simulink model "GPS1_Kvaser_R2018a_v3_0719"  (R2018a)
settings: Solver=FixedStepAuto  StartTime=0.0  StopTime=inf  FixedStep=0.02  RelTol=1e-3
undefined symbols (not defined in the file): canChannel
libraries: dspinverses x11, canmsglib x6, canlib x4
(part 1 of 2)
settings Model: Creator=ZNYZY  LastModifiedBy=RickyFang
settings SFSimCC: SimUseLocalCustomCode=on
settings RTWCC: RTWUseLocalCustomCode=on

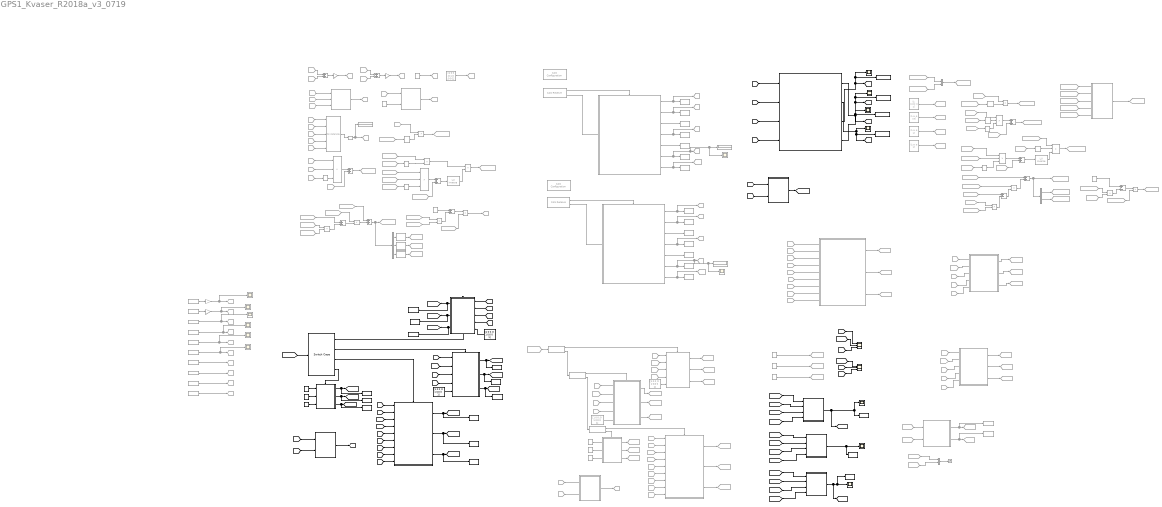
== system GPS1_Kvaser_R2018a_v3_0719 ==
  note: head要乘pi/180
  note: 离线仿真
  note: 试验设计
      | 1.双GPS走同一直线，改L值，反复3次
      | 2.双GPS贴在一起，改L值，反复3次
      | 3.双GPS走同一段曲线，改L值，反复3次
  note: 最终用于EKF卡尔曼滤波的观测速度
  note: dSPACE
  note: 通道1：GPS1的信号——取sate1、head1、lat1、long1、speed1
      | 通道2：GPS2的信号——取sate2、head2、lat2、long2、speed2
      | 通道3：车辆信号——取Vehicle_Speed、Acc_Ego
  note: EKF_mode = 3
  note: GPS测得车速与车身DBC的车速进行比较选择
  note: X_predict = A*X_optimal(:,i-1);
  note: EKF_mode=3，单GPS2工作；
      | EKF_mode=2，单GPS1工作；
      | EKF_mode=1，双GPS融合工作；
      | EKF_mode=0，不可测；
  note: 得到EKF的模式
  note: GPS经纬度坐标系转大地坐标系
  note: Kvaser读取GPS
  note: EKF_mode = 1
  note: EKF_mode = 2
  note: EKF_mode = 0
  note: EKF_mode = 3
  note: EKF_mode = 1
  note: EKF_mode = 0.1.2
  note: EKF_mode = 2
  note: EKF_mode = 1
  note: EKF_mode = 0
  note: EKF_mode判断逻辑
  note: EKF_mode判断逻辑
  " LU Inverse" : dspinverses/ LU Inverse  Commented=on
  " LU Inverse1" : dspinverses/ LU Inverse  Commented=on
  Add : Sum  Commented=on  Inputs=+-
  CAN Configuration : canlib/CAN Configuration  Commented=on  BlockHandle=4516.0012  Device=MathWorks Virtual 1 (Channel 1)  DeviceMenu=MathWorks Virtual 1 (Channel 1)  ObjConstructor=canChannel('MathWorks', 'Virtual 1', 1)  BusSpeed=500000  EnableBitParameters=off  AckMode=Normal
      settings: SourceProductBaseCode=VN
  CAN Configuration1 : canlib/CAN Configuration  Commented=on  BlockHandle=4517.0012  Device=MathWorks Virtual 1 (Channel 1)  DeviceMenu=MathWorks Virtual 1 (Channel 1)  ObjConstructor=canChannel('MathWorks', 'Virtual 1', 1)  BusSpeed=500000  EnableBitParameters=off  AckMode=Normal
      settings: SourceProductBaseCode=VN
  CAN Receive1 : canlib/CAN Receive  Commented=on  BlockHandle=4518.0012  Device=MathWorks Virtual 1 (Channel 1)  DeviceMenu=MathWorks Virtual 1 (Channel 1)  ObjConstructor=canChannel('MathWorks', 'Virtual 1', 1)  EnableStandardIDsFilter=off  StdIDsCombo=Allow all  StandardIDs=0  EnableExtendedIDsFilter=off  ExtIDsCombo=Allow all  ExtendedIDs=0  SampleTime=0.01  MsgsPerTimestep=all  InternalFilterUpdateStatus=on  BusOutput=off
      settings: SourceProductBaseCode=VN
  CAN Receive2 : canlib/CAN Receive  Commented=on  BlockHandle=4519.0012  Device=MathWorks Virtual 1 (Channel 1)  DeviceMenu=MathWorks Virtual 1 (Channel 1)  ObjConstructor=canChannel('MathWorks', 'Virtual 1', 1)  EnableStandardIDsFilter=off  StdIDsCombo=Allow all  StandardIDs=0  EnableExtendedIDsFilter=off  ExtIDsCombo=Allow all  ExtendedIDs=0  SampleTime=0.01  MsgsPerTimestep=all  InternalFilterUpdateStatus=on  BusOutput=off
      settings: SourceProductBaseCode=VN
  Constant : Constant  Commented=on  Value=[1 0 0 ;0 1 0 ;0 0 1]
  Constant1 : Constant  Commented=on  Value=0.01
  Constant{4..7,10..11} (6 alike) : Constant  Commented=on  Value=0
  Constant12 : Constant  Commented=on  Value=[1 0 0 ;0 1 0;0 0 1]
  Constant13 : Constant  Value=0
  Constant14 : Constant  Value=[1 0 0 ;0 1 0;0 0 1]
  Constant15 : Constant  Value=0
  Constant16 : Constant  Value=[1 0 0 ;0 1 0;0 0 1]
  Constant17 : Constant  Commented=on  Value=[1 0.02; 0 1]
  Constant18 : Constant  Commented=on  Value=[1 0; 0 10]
  Constant19 : Constant  Commented=on  Value=[1 0; 0 1]
  Constant2 : Constant  Commented=on  Value=0.3
  Constant20 : Constant  Commented=on  Value=[1 0; 0 1]
  Constant21 : Constant  Commented=on  Value=eye(2)
  Constant3 : Constant  Commented=on  Value=eye(3)
  Constant8 : Constant  Value=0
  Constant9 : Constant  Commented=on  Value=[1 0 0 ;0 1 0;0 0 1]
  Delay : Delay  Commented=on  DelayLength=1
  Delay1 : Delay  Commented=on  DelayLength=1
  Delay2 : Delay  Commented=on  DelayLength=1
  Demux : Demux  Commented=on  Outputs=3
  Demux1 : Demux  Commented=on  Outputs=2
  Display : Display  Commented=on
  Display1 : Display  Commented=on
  Display2 : Display  Commented=on
  EKF_HEAD : Scope
  EKF_HEAD_SUB : Subsystem
  EKF_LAT : Scope
  EKF_LAT_SUB : Subsystem
  EKF_LONG : Scope
  EKF_LONG_SUB : Subsystem
  From Workspace : FromWorkspace  Commented=on  VariableName=head1
  From Workspace1 : FromWorkspace  Commented=on  VariableName=head2
  From Workspace2 : FromWorkspace  Commented=on  VariableName=lat1
  From Workspace3 : FromWorkspace  Commented=on  VariableName=lat2
  From Workspace4 : FromWorkspace  Commented=on  VariableName=long1
  From Workspace5 : FromWorkspace  Commented=on  VariableName=long2
  From Workspace6 : FromWorkspace  Commented=on  VariableName=sate1
  From Workspace7 : FromWorkspace  Commented=on  VariableName=sate2
  From Workspace8 : FromWorkspace  Commented=on  VariableName=speed1
  From Workspace9 : FromWorkspace  Commented=on  VariableName=speed2
  From{10,15,18,65,77,133} (6 alike) : From  Commented=on  GotoTag=speed1
  From11 : From  Commented=on  GotoTag=long1
  From110 : From  Commented=on  GotoTag=Vehicle_Speed
  From111 : From  Commented=on  GotoTag=Acc_Ego
  From112 : From  Commented=on  GotoTag=X_optimal_vehicle
  From113 : From  Commented=on  GotoTag=A_Vehicle
  From114 : From  Commented=on  GotoTag=A_Vehicle
  From115 : From  Commented=on  GotoTag=A_Vehicle
  From116 : From  Commented=on  GotoTag=P_Vehicle
  From117 : From  Commented=on  GotoTag=Q_Vehicle
  From{118,120,122,127,130} (5 alike) : From  Commented=on  GotoTag=C_Vehicle
  From119 : From  Commented=on  GotoTag=P_predict_Vehicle
  From{9,12,16,73..74} (5 alike) : From  Commented=on  GotoTag=head1
  From121 : From  Commented=on  GotoTag=P_predict_Vehicle
  From123 : From  Commented=on  GotoTag=R_Vehicle
  From124 : From  Commented=on  GotoTag=X_predict_vehicle
  From125 : From  Commented=on  GotoTag=K_Vehicle
  From126 : From  Commented=on  GotoTag=Y_Vehicle
  From128 : From  Commented=on  GotoTag=X_predict_vehicle
  From129 : From  Commented=on  GotoTag=K_Vehicle
  From13 : From  Commented=on  GotoTag=long1
  From131 : From  Commented=on  GotoTag=P_predict_Vehicle
  From132 : From  Commented=on  GotoTag=KF_Vehicle_Speed
  From{19,50,54,61,69,134} (6 alike) : From  Commented=on  GotoTag=speed2
  From135 : From  Commented=on  GotoTag=sate1
  From136 : From  Commented=on  GotoTag=sate2
  From137 : From  Commented=on  GotoTag=EKF_lat
  From138 : From  Commented=on  GotoTag=EKF_long
  From139 : From  Commented=on  GotoTag=EKF_long_abs
  From14 : From  Commented=on  GotoTag=lat1
  From140 : From  Commented=on  GotoTag=EKF_lat_abs
  From{7,17,53,63,68} (5 alike) : From  Commented=on  GotoTag=head2
  From20 : From  Commented=on  GotoTag=y2
  From21 : From  Commented=on  GotoTag=y1
  From22 : From  Commented=on  GotoTag=x2
  From23 : From  Commented=on  GotoTag=x1
  From24 : From  Commented=on
  From25 : From  Commented=on  GotoTag=X_optimal
  From26 : From  Commented=on
  From27 : From  Commented=on  GotoTag=P
  From28 : From  Commented=on
  From29 : From  Commented=on  GotoTag=Q
  From30 : From  Commented=on  GotoTag=P_predict
  From{31..32,34,39,42} (5 alike) : From  Commented=on  GotoTag=C
  From33 : From  Commented=on  GotoTag=P_predict
  From{6,35,51,57,72} (5 alike) : From  Commented=on  GotoTag=R
  From36 : From  Commented=on  GotoTag=X_predict
  From37 : From  Commented=on  GotoTag=K
  From38 : From  Commented=on  GotoTag=Y
  From40 : From  Commented=on  GotoTag=X_predict
  From41 : From  Commented=on  GotoTag=K
  From43 : From  Commented=on  GotoTag=P_predict
  From44 : From  Commented=on  GotoTag=head
  From45 : From  Commented=on  GotoTag=speed
  From46 : From  Commented=on  GotoTag=T
  From47 : From  Commented=on  GotoTag=head
  From48 : From  Commented=on  GotoTag=head
  From49 : From  Commented=on  GotoTag=lat2
  From52 : From  Commented=on  GotoTag=lat1
  From55 : From  Commented=on  GotoTag=long2
  From56 : From  Commented=on  GotoTag=lat2
  From58 : From  Commented=on  GotoTag=x1
  From59 : From  Commented=on  GotoTag=EKF_mode
  From60 : From  Commented=on  GotoTag=x2
  From62 : From  Commented=on  GotoTag=sate1
  From64 : From  Commented=on  GotoTag=y2
  From75 : From  Commented=on  GotoTag=y1
  From76 : From  Commented=on  GotoTag=x1
  From78 : From  Commented=on  GotoTag=sate2
  From79 : From  Commented=on  GotoTag=x2
  From8 : From  Commented=on  GotoTag=long2
  From80 : From  Commented=on  GotoTag=y1
  From81 : From  Commented=on  GotoTag=y2
  Function-Call Subsystem1 : Subsystem  Commented=on  TreatAsAtomicUnit=on
  Function-Call Subsystem2 : Subsystem  Commented=on  TreatAsAtomicUnit=on
  Gain : Gain  Commented=on  Gain=0.5
  Gain1 : Gain  Commented=on  Gain=0.5
  Gain2 : Gain  Commented=on  Gain=pi/180
  Gain3 : Gain  Commented=on  Gain=pi/180
  Goto : Goto  Commented=on  GotoTag=lat1
  Goto1 : Goto  Commented=on  GotoTag=long1
  Goto10 : Goto  Commented=on  GotoTag=head2
  Goto12 : Goto  Commented=on  GotoTag=sate2
  Goto13 : Goto  Commented=on  GotoTag=speed2
  Goto2 : Goto  Commented=on  GotoTag=R
  Goto20 : Goto  Commented=on  GotoTag=head
  Goto21 : Goto  Commented=on  GotoTag=speed
  Goto22 : Goto  Commented=on  GotoTag=T
  Goto23 : Goto  Commented=on
  Goto24 : Goto  Commented=on  GotoTag=C
  Goto25 : Goto  Commented=on  GotoTag=Y
  Goto26 : Goto  Commented=on  GotoTag=X_predict
  Goto27 : Goto  Commented=on  GotoTag=P_predict
  Goto28 : Goto  Commented=on  GotoTag=K
  Goto29 : Goto  Commented=on  GotoTag=P
  Goto3 : Goto  Commented=on  GotoTag=head1
  Goto30 : Goto  Commented=on  GotoTag=X_optimal
  Goto31 : Goto  Commented=on  GotoTag=Q
  Goto32 : Goto  Commented=on  GotoTag=EKF_lat1
  Goto33 : Goto  Commented=on  GotoTag=EKF_long1
  Goto34 : Goto  Commented=on  GotoTag=EKF_head1
  Goto35 : Goto  Commented=on  GotoTag=EKF_lat3
  Goto36 : Goto  Commented=on  GotoTag=EKF_long3
  Goto37 : Goto  Commented=on  GotoTag=EKF_head3
  Goto38 : Goto  Commented=on  GotoTag=EKF_lat1
  Goto39 : Goto  Commented=on  GotoTag=EKF_long1
  Goto40 : Goto  Commented=on  GotoTag=EKF_head1
  Goto41 : Goto  Commented=on  GotoTag=EKF_lat0
  Goto42 : Goto  Commented=on  GotoTag=EKF_long0
  Goto43 : Goto  Commented=on  GotoTag=EKF_head0
  Goto44 : Goto  Commented=on  GotoTag=EKF_lat3
  Goto45 : Goto  Commented=on  GotoTag=EKF_long3
  Goto46 : Goto  Commented=on  GotoTag=EKF_head3
  Goto47 : Goto  Commented=on  GotoTag=EKF_lat0
  Goto48 : Goto  Commented=on  GotoTag=EKF_long0
  Goto49 : Goto  Commented=on  GotoTag=EKF_head0
  Goto5 : Goto  Commented=on  GotoTag=sate1
  Goto50 : Goto  Commented=on  GotoTag=EKF_lat2
  Goto51 : Goto  Commented=on  GotoTag=EKF_long2
  Goto52 : Goto  Commented=on  GotoTag=EKF_head2
  Goto53 : Goto  Commented=on  GotoTag=EKF_lat1
  Goto54 : Goto  Commented=on  GotoTag=EKF_long1
  Goto55 : Goto  Commented=on  GotoTag=EKF_head1
  Goto56 : Goto  Commented=on  GotoTag=EKF_lat2
  Goto57 : Goto  Commented=on  GotoTag=EKF_long2
  Goto58 : Goto  Commented=on  GotoTag=EKF_head2
  Goto6 : Goto  Commented=on  GotoTag=speed1
  Goto68 : Goto  Commented=on  GotoTag=Y_Vehicle
  Goto69 : Goto  Commented=on  GotoTag=A_Vehicle
  Goto7 : Goto  Commented=on  GotoTag=lat2
  Goto70 : Goto  Commented=on  GotoTag=R_Vehicle
  Goto71 : Goto  Commented=on  GotoTag=Q_Vehicle
  Goto72 : Goto  Commented=on  GotoTag=C_Vehicle
  Goto73 : Goto  Commented=on  GotoTag=P_Vehicle
  Goto74 : Goto  Commented=on  GotoTag=X_predict_vehicle
  Goto75 : Goto  Commented=on  GotoTag=P_predict_Vehicle
  Goto76 : Goto  Commented=on  GotoTag=K_Vehicle
  Goto77 : Goto  Commented=on  GotoTag=X_optimal_vehicle
  Goto78 : Goto  Commented=on  GotoTag=KF_Vehicle_Speed
  Goto79 : Goto  Commented=on  GotoTag=KF_Acc_Ego
  Goto8 : Goto  Commented=on  GotoTag=long2
  Goto80 : Goto  Commented=on  GotoTag=speed_end
  Goto84 : Goto  Commented=on  GotoTag=head1
  Goto85 : Goto  Commented=on  GotoTag=EKF_long_abs
  Goto86 : Goto  Commented=on  GotoTag=EKF_lat_abs
  Goto87 : Goto  Commented=on  GotoTag=head2
  Goto88 : Goto  Commented=on  GotoTag=lat1
  Goto89 : Goto  Commented=on  GotoTag=lat2
  Goto90 : Goto  Commented=on  GotoTag=long1
  Goto91 : Goto  Commented=on  GotoTag=long2
  Goto92 : Goto  Commented=on  GotoTag=sate1
  Goto93 : Goto  Commented=on  GotoTag=sate2
  Goto94 : Goto  Commented=on  GotoTag=speed1
  Goto95 : Goto  Commented=on  GotoTag=speed2
  If Action Subsystem1 : Subsystem  Commented=on  TreatAsAtomicUnit=on
  If Action Subsystem2 : Subsystem  TreatAsAtomicUnit=on
  If Action Subsystem3 : Subsystem  Commented=on  TreatAsAtomicUnit=on
  If Action Subsystem4 : Subsystem  Commented=on  TreatAsAtomicUnit=on
  If Action Subsystem5 : Subsystem  Commented=on  TreatAsAtomicUnit=on
  If Action Subsystem6 : Subsystem  TreatAsAtomicUnit=on
  If Action Subsystem7 : Subsystem  TreatAsAtomicUnit=on
  If Action Subsystem8 : Subsystem  TreatAsAtomicUnit=on
  If1 : If  Commented=on  IfExpression=u1 > 2
  If2 : If  Commented=on  IfExpression=u1 > 1
  If3 : If  Commented=on
  MATLAB Function : MATLAB Function  TreatAsAtomicUnit=on
  MATLAB Function1 : MATLAB Function  TreatAsAtomicUnit=on
  MATLAB Function2 : MATLAB Function  Commented=on  TreatAsAtomicUnit=on
  MATLAB Function3 : MATLAB Function  Commented=on  TreatAsAtomicUnit=on
  MATLAB Function4 : MATLAB Function  Commented=on  TreatAsAtomicUnit=on
  MATLAB Function5 : MATLAB Function  TreatAsAtomicUnit=on
  MATLAB Function6 : MATLAB Function  Commented=on  TreatAsAtomicUnit=on
  MATLAB Function7 : MATLAB Function  Commented=on  TreatAsAtomicUnit=on
  Matrix Concatenate : Concatenate  Commented=on  NumInputs=5  Mode=Multidimensional array  ConcatenateDimension=2
  Mux : Mux  Commented=on  Inputs=2
  Mux1 : Mux  Commented=on  Inputs=2
  Plus{,1..4,10..11,13} (8 alike) : Sum  Commented=on
  Plus12 : Sum  Commented=on  Inputs=+-
  Plus5 : Sum  Commented=on  Inputs=+-
  Plus6 : Sum  Commented=on  Inputs=+-
  Product{,3..9,13..16} (12 alike) : Product  Commented=on
  Product{1..2,10..12} (5 alike) : Product  Commented=on  Inputs=3
  Reshape : Reshape  Commented=on  OutputDimensionality=Customize  OutputDimensions=[4,1]
  Scope{3..10} (8 alike) : Scope  Commented=on
  Scope{11..14} (4 alike) : Scope
  Scope15 : Scope  NumInputPorts=3
  Scope16 : Scope  NumInputPorts=3
  Subsystem : Subsystem  Commented=on
  Subsystem1 : Subsystem  Commented=on
  Subsystem2 : Subsystem  Commented=on
  Subsystem3 : Subsystem  Commented=on
  Subsystem4 : Subsystem  Commented=on
  Subsystem6 : Subsystem  Commented=on
  Switch Case : SwitchCase  CaseConditions={3,2,1}
  Terminator : Terminator  Commented=on
  To Workspace : ToWorkspace  Commented=on  VariableName=EKF_lat_abs  SampleTime=-1
  To Workspace1 : ToWorkspace  VariableName=EKF_head  SampleTime=-1
  To Workspace10 : ToWorkspace  Commented=on  VariableName=speed1  SampleTime=-1
  To Workspace11 : ToWorkspace  VariableName=EKF_head1  SampleTime=-1
  To Workspace12 : ToWorkspace  VariableName=EKF_long1  SampleTime=-1
  To Workspace13 : ToWorkspace  VariableName=EKF_lat2  SampleTime=-1
  To Workspace14 : ToWorkspace  Commented=on  VariableName=speed2  SampleTime=-1
  To Workspace15 : ToWorkspace  Commented=on  VariableName=lat2  SampleTime=-1
  To Workspace16 : ToWorkspace  Commented=on  VariableName=long2  SampleTime=-1
  To Workspace17 : ToWorkspace  Commented=on  VariableName=al2  SampleTime=-1
  To Workspace18 : ToWorkspace  Commented=on  VariableName=head2  SampleTime=-1
  To Workspace19 : ToWorkspace  Commented=on  VariableName=position_type2  SampleTime=-1
  To Workspace2 : ToWorkspace  Commented=on  VariableName=EKF_long_abs  SampleTime=-1
  To Workspace20 : ToWorkspace  Commented=on  VariableName=sate2  SampleTime=-1
  To Workspace21 : ToWorkspace  VariableName=EKF_head2  SampleTime=-1
  To Workspace22 : ToWorkspace  VariableName=EKF_long2  SampleTime=-1
  To Workspace23 : ToWorkspace  VariableName=EKF_lat3  SampleTime=-1
  To Workspace24 : ToWorkspace  VariableName=EKF_long3  SampleTime=-1
  To Workspace25 : ToWorkspace  VariableName=EKF_head3  SampleTime=-1
  To Workspace26 : ToWorkspace  VariableName=EKF_lat0  SampleTime=-1
  To Workspace27 : ToWorkspace  VariableName=EKF_long0  SampleTime=-1
  To Workspace28 : ToWorkspace  VariableName=EKF_head0  SampleTime=-1
  To Workspace29 : ToWorkspace  VariableName=EKF_lat_abs  SampleTime=-1
  To Workspace3 : ToWorkspace  VariableName=EKF_lat1  SampleTime=-1
  To Workspace30 : ToWorkspace  VariableName=EKF_long_abs  SampleTime=-1
  To Workspace31 : ToWorkspace  VariableName=x1  SampleTime=-1
  To Workspace32 : ToWorkspace  VariableName=x2  SampleTime=-1
  To Workspace33 : ToWorkspace  VariableName=y1  SampleTime=-1
  To Workspace34 : ToWorkspace  VariableName=y2  SampleTime=-1
  To Workspace4 : ToWorkspace  Commented=on  VariableName=lat1  SampleTime=-1
  To Workspace5 : ToWorkspace  Commented=on  VariableName=long1  SampleTime=-1
  To Workspace6 : ToWorkspace  Commented=on  VariableName=al1  SampleTime=-1
  To Workspace7 : ToWorkspace  Commented=on  VariableName=head1  SampleTime=-1
  To Workspace8 : ToWorkspace  Commented=on  VariableName=position_type1  SampleTime=-1
  To Workspace9 : ToWorkspace  Commented=on  VariableName=sate1  SampleTime=-1
  Transpose{,1..5} (6 alike) : Math  Commented=on  Operator=transpose  SaturateOnIntegerOverflow=on
  wires:
  Function-Call Subsystem1/1(Out1) -> Goto/1, To Workspace4/1
  Function-Call Subsystem1/2(Out2) -> Goto1/1, To Workspace5/1
  Function-Call Subsystem1/3(Out3) -> To Workspace6/1
  Function-Call Subsystem1/4(Out4) -> Goto3/1, To Workspace7/1
  CAN Receive1/1 -> Function-Call Subsystem1/Trigger
  CAN Receive1/2 -> Function-Call Subsystem1/1(In1)
  Function-Call Subsystem1/6(Out6) -> Scope4/1, Display1/1, Goto5/1, To Workspace9/1
  Function-Call Subsystem1/5(Out5) -> To Workspace8/1
  Function-Call Subsystem1/7(Out7) -> Goto6/1, To Workspace10/1
  Function-Call Subsystem2/6(Out6) -> Scope3/1, Display2/1, Goto12/1, To Workspace20/1
  Function-Call Subsystem2/5(Out5) -> To Workspace19/1
  Function-Call Subsystem2/7(Out7) -> Goto13/1, To Workspace14/1
  Function-Call Subsystem2/4(Out4) -> Goto10/1, To Workspace18/1
  Function-Call Subsystem2/2(Out2) -> Goto8/1, To Workspace16/1
  CAN Receive2/2 -> Function-Call Subsystem2/1(In1)
  CAN Receive2/1 -> Function-Call Subsystem2/Trigger
  Function-Call Subsystem2/1(Out1) -> Goto7/1, To Workspace15/1
  Function-Call Subsystem2/3(Out3) -> To Workspace17/1
  [lat1] -> MATLAB Function/1(lat1)
  [long1] -> MATLAB Function/3(long1)
  [long2] -> MATLAB Function/4(long2)
  [lat2] -> MATLAB Function/2(lat2)
  MATLAB Function/3(dikaerX1) -> To Workspace31/1, Scope11/1, [x1]
  MATLAB Function/2(dikaerY2) -> [y2], To Workspace34/1, Scope14/1
  MATLAB Function/1(dikaerY1) -> [y1], To Workspace33/1, Scope13/1
  [sate1] -> MATLAB Function1/2(sate2)
  [sate2] -> MATLAB Function1/1(sate1)
  MATLAB Function1/1(EKF_mode) -> [EKF_mode]
  Plus/1 -> Gain/1
  From17/1 -> Plus/2
  From16/1 -> Plus/1
  Gain/1 -> Goto20/1
  Gain1/1 -> Goto21/1
  Plus1/1 -> Gain1/1
  From19/1 -> Plus1/2
  From18/1 -> Plus1/1
  Constant1/1 -> Goto22/1
  MATLAB Function3/1(A) -> Goto23/1
  MATLAB Function4/1(C) -> Goto24/1
  From23/1 -> Matrix Concatenate/1
  From22/1 -> Matrix Concatenate/2
  From21/1 -> Matrix Concatenate/3
  From20/1 -> Matrix Concatenate/4
  Matrix Concatenate/1 -> Reshape/1
  Reshape/1 -> Goto25/1, Display/1
  From25/1 -> Delay/1
  Delay/1 -> Product/2
  From24/1 -> Product/1
  Product/1 -> Goto26/1
  From28/1 -> Transpose/1
  Transpose/1 -> Product1/3
  From26/1 -> Product1/1
  From27/1 -> Product1/2
  Product1/1 -> Plus2/1
  From29/1 -> Plus2/2
  Plus2/1 -> Goto27/1
  From31/1 -> Transpose1/1
  From34/1 -> Transpose2/1
  Transpose2/1 -> Product2/3
  From33/1 -> Product2/2
  From32/1 -> Product2/1
  Product2/1 -> Plus3/1
  From35/1 -> Plus3/2
  Plus3/1 -> " LU Inverse"/1
  Transpose1/1 -> Product4/2
  From30/1 -> Product4/1
  Product4/1 -> Product3/1
  " LU Inverse"/1 -> Product3/2
  Product3/1 -> Goto28/1
  From39/1 -> Product5/1
  From40/1 -> Product5/2
  Product5/1 -> Plus5/2
  From38/1 -> Plus5/1
  Plus5/1 -> Product6/2
  From37/1 -> Product6/1
  Product6/1 -> Plus4/2
  From36/1 -> Plus4/1
  Plus4/1 -> Demux/1, Goto30/1
  Constant3/1 -> Plus6/1
  From41/1 -> Product7/1
  From42/1 -> Product7/2
  Product7/1 -> Plus6/2
  Plus6/1 -> Product8/1
  From43/1 -> Product8/2
  Product8/1 -> Goto29/1
  From44/1 -> MATLAB Function3/1(theta)
  From45/1 -> MATLAB Function3/2(v)
  From46/1 -> MATLAB Function3/3(T)
  Constant/1 -> Goto31/1
  From47/1 -> MATLAB Function4/1(theta)
  Constant2/1 -> MATLAB Function4/2(L)
  Demux/1 -> Subsystem/1(In1)
  Demux/2 -> Subsystem1/1(In1)
  Demux/3 -> Subsystem2/1(In1)
  Constant5/1 -> Goto42/1
  Constant4/1 -> Goto41/1
  Constant6/1 -> Goto43/1
  Subsystem/1(Out1) -> Goto32/1
  Subsystem1/1(Out1) -> Goto33/1
  Subsystem2/1(Out1) -> Goto34/1
  Subsystem6/1(Out1) -> Goto50/1
  Subsystem6/2(Out2) -> Goto51/1
  Subsystem6/3(Out3) -> Goto52/1
  From12/1 -> Subsystem6/1(In1)
  From14/1 -> Subsystem6/3(In3)
  From13/1 -> Subsystem6/4(In4)
  From15/1 -> Subsystem6/2(In2)
  From48/1 -> Matrix Concatenate/5
  From6/1 -> Subsystem6/5(In5)
  Subsystem3/3(Out3) -> Goto37/1
  From51/1 -> Subsystem3/5(In5)
  From49/1 -> Subsystem3/3(In3)
  From7/1 -> Subsystem3/1(In1)
  Subsystem3/1(Out1) -> Goto35/1
  From50/1 -> Subsystem3/2(In2)
  Subsystem3/2(Out2) -> Goto36/1
  From8/1 -> Subsystem3/4(In4)
  Subsystem4/3(Out3) -> Goto40/1
  Subsystem4/2(Out2) -> Goto39/1
  Subsystem4/1(Out1) -> Goto38/1
  From56/1 -> Subsystem4/6(x2)
  From55/1 -> Subsystem4/8(y2)
  From10/1 -> Subsystem4/3(speed1)
  From11/1 -> Subsystem4/7(y1)
  From52/1 -> Subsystem4/5(x1)
  From9/1 -> Subsystem4/1(head1)
  From54/1 -> Subsystem4/4(speed2)
  From53/1 -> Subsystem4/2(head2)
  From57/1 -> Subsystem4/9(R)
  From59/1 -> If1/1
  If1/1 -> If Action Subsystem1/Action
  If1/2 -> If2/1
  If2/1 -> If Action Subsystem3/Action
  If2/2 -> If3/1
  If3/1 -> If Action Subsystem4/Action
  If3/2 -> If Action Subsystem5/Action
  From61/1 -> If Action Subsystem1/2(In2)
  From64/1 -> If Action Subsystem1/4(In4)
  From63/1 -> If Action Subsystem1/1(In1)
  Constant12/1 -> If Action Subsystem1/5(In5)
  From60/1 -> If Action Subsystem1/3(In3)
  If Action Subsystem1/2(Out2) -> Goto45/1
  If Action Subsystem1/3(Out3) -> Goto46/1
  If Action Subsystem1/1(Out1) -> Goto44/1
  Constant7/1 -> If Action Subsystem5/1(In1)
  Constant10/1 -> If Action Subsystem5/2(In2)
  Constant11/1 -> If Action Subsystem5/3(In3)
  If Action Subsystem5/1(Out1) -> Goto47/1
  If Action Subsystem5/2(Out2) -> Goto48/1
  If Action Subsystem5/3(Out3) -> Goto49/1
  From58/1 -> If Action Subsystem4/5(x1)
  From80/1 -> If Action Subsystem4/7(y1)
  From81/1 -> If Action Subsystem4/8(y2)
  From65/1 -> If Action Subsystem4/3(speed1)
  From72/1 -> If Action Subsystem4/9(R)
  From79/1 -> If Action Subsystem4/6(x2)
  From69/1 -> If Action Subsystem4/4(speed2)
  From68/1 -> If Action Subsystem4/2(head2)
  From73/1 -> If Action Subsystem4/1(head1)
  If Action Subsystem4/2(Out2) -> Goto54/1
  If Action Subsystem4/3(Out3) -> Goto55/1
  If Action Subsystem4/1(Out1) -> Goto53/1
  Constant9/1 -> If Action Subsystem3/5(In5)
  From76/1 -> If Action Subsystem3/3(In3)
  From74/1 -> If Action Subsystem3/1(In1)
  From77/1 -> If Action Subsystem3/2(In2)
  From75/1 -> If Action Subsystem3/4(In4)
  If Action Subsystem3/1(Out1) -> Goto56/1
  If Action Subsystem3/2(Out2) -> Goto57/1
  If Action Subsystem3/3(Out3) -> Goto58/1
  From62/1 -> MATLAB Function2/1(sate1)
  MATLAB Function2/1(R) -> Goto2/1
  From78/1 -> MATLAB Function2/2(sate2)
  [sate2] -> MATLAB Function5/2(sate2)
  Constant14/1 -> If Action Subsystem2/5(In5)
  [sate1] -> MATLAB Function5/1(sate1)
  Constant8/1 -> If Action Subsystem8/2(In2)
  [R] -> If Action Subsystem7/9(R)
  [y2] -> If Action Subsystem2/4(In4)
  [y1] -> If Action Subsystem6/4(In4)
  [speed2] -> If Action Subsystem7/4(speed2)
  Switch Case/2 -> If Action Subsystem6/Action
  If Action Subsystem7/3(Out3) -> To Workspace11/1, [EKF_head1]
  [speed1] -> If Action Subsystem6/2(In2)
  [speed2] -> If Action Subsystem2/2(In2)
  [x1] -> If Action Subsystem6/3(In3)
  [x2] -> If Action Subsystem7/6(x2)
  [speed1] -> If Action Subsystem7/3(speed1)
  Constant16/1 -> If Action Subsystem6/5(In5)
  [y2] -> If Action Subsystem7/8(y2)
  [x1] -> If Action Subsystem7/5(x1)
  [y1] -> If Action Subsystem7/7(y1)
  Switch Case/4 -> If Action Subsystem8/Action
  If Action Subsystem8/3(Out3) -> To Workspace28/1, [EKF_head0]
  If Action Subsystem2/3(Out3) -> To Workspace25/1, [EKF_head3]
  Constant15/1 -> If Action Subsystem8/1(In1)
  [EKF_mode] -> Switch Case/1
  [head1] -> If Action Subsystem6/1(In1)
  If Action Subsystem6/3(Out3) -> To Workspace21/1, [EKF_head2]
  [x2] -> If Action Subsystem2/3(In3)
  MATLAB Function5/1(R) -> [R]
  Constant13/1 -> If Action Subsystem8/3(In3)
  [head2] -> If Action Subsystem2/1(In1)
  Switch Case/1 -> If Action Subsystem2/Action
  [head1] -> If Action Subsystem7/1(head1)
  [head2] -> If Action Subsystem7/2(head2)
  Switch Case/3 -> If Action Subsystem7/Action
  From110/1 -> Mux/1
  From111/1 -> Mux/2
  Mux/1 -> Goto68/1
  Constant17/1 -> Goto69/1
  Constant18/1 -> Goto70/1
  Constant19/1 -> Goto71/1
  Constant20/1 -> Goto72/1
  From112/1 -> Delay1/1
  Delay1/1 -> Product9/2
  From113/1 -> Product9/1
  Product9/1 -> Goto74/1
  From115/1 -> Transpose3/1
  From116/1 -> Delay2/1
  Transpose3/1 -> Product10/3
  From114/1 -> Product10/1
  Product10/1 -> Plus10/1
  From117/1 -> Plus10/2
  Plus10/1 -> Goto75/1
  From118/1 -> Transpose4/1
  From122/1 -> Transpose5/1
  From121/1 -> Product11/2
  From120/1 -> Product11/1
  Transpose5/1 -> Product11/3
  Product11/1 -> Plus11/1
  From123/1 -> Plus11/2
  Plus11/1 -> " LU Inverse1"/1
  " LU Inverse1"/1 -> Product12/3
  Transpose4/1 -> Product12/2
  From119/1 -> Product12/1
  Product12/1 -> Goto76/1
  Delay2/1 -> Product10/2
  From127/1 -> Product13/1
  From128/1 -> Product13/2
  From126/1 -> Plus12/1
  Product13/1 -> Plus12/2
  From125/1 -> Product14/1
  Plus12/1 -> Product14/2
  From124/1 -> Plus13/1
  Product14/1 -> Plus13/2
  Plus13/1 -> Demux1/1, Goto77/1
  From129/1 -> Product15/1
  From130/1 -> Product15/2
  Constant21/1 -> Add/1
  Product15/1 -> Add/2
  Add/1 -> Product16/1
  From131/1 -> Product16/2
  Product16/1 -> Goto73/1
  Demux1/2 -> Goto79/1
  Demux1/1 -> Goto78/1
  From136/1 -> MATLAB Function6/5(sate2)
  From134/1 -> MATLAB Function6/3(speed2)
  From135/1 -> MATLAB Function6/4(sate1)
  From133/1 -> MATLAB Function6/2(speed1)
  From132/1 -> MATLAB Function6/1(kf_vehicle_speed)
  MATLAB Function6/1(speed_end) -> Goto80/1
  If Action Subsystem7/2(Out2) -> To Workspace3/1, [EKF_lat1]
  If Action Subsystem7/1(Out1) -> To Workspace12/1, [EKF_long1]
  If Action Subsystem6/1(Out1) -> To Workspace22/1, [EKF_long2]
  If Action Subsystem6/2(Out2) -> [EKF_lat2], To Workspace13/1
  If Action Subsystem2/2(Out2) -> [EKF_lat3], To Workspace23/1
  If Action Subsystem2/1(Out1) -> [EKF_long3], To Workspace24/1
  If Action Subsystem8/2(Out2) -> To Workspace26/1, [EKF_lat0]
  If Action Subsystem8/1(Out1) -> [EKF_long0], To Workspace27/1
  From138/1 -> MATLAB Function7/1(long1)
  From137/1 -> MATLAB Function7/2(lat1)
  MATLAB Function7/1(A_x1) -> To Workspace2/1, Goto85/1
  MATLAB Function7/2(A_y1) -> To Workspace/1, Goto86/1
  From139/1 -> Mux1/1
  From140/1 -> Mux1/2
  Mux1/1 -> Terminator/1
  From Workspace/1 -> Gain2/1
  From Workspace1/1 -> Gain3/1
  From Workspace2/1 -> Scope7/1, Goto88/1
  From Workspace3/1 -> Scope8/1, Goto89/1
  From Workspace4/1 -> Scope9/1, Goto90/1
  From Workspace5/1 -> Scope10/1, Goto91/1
  From Workspace6/1 -> Goto92/1
  From Workspace7/1 -> Goto93/1
  From Workspace8/1 -> Goto94/1
  From Workspace9/1 -> Goto95/1
  Gain2/1 -> Scope5/1, Goto84/1
  Gain3/1 -> Scope6/1, Goto87/1
  MATLAB Function/4(dikaerX2) -> To Workspace32/1, Scope12/1, [x2]
  [EKF_long] -> Scope15/2
  [x1] -> Scope15/3
  [x2] -> Scope15/1
  [y1] -> Scope16/2
  [EKF_lat] -> Scope16/1
  [y2] -> Scope16/3
  EKF_LAT_SUB/1(EKF_LAT) -> [EKF_lat], To Workspace30/1, EKF_LAT/1
  [EKF_lat3] -> EKF_LAT_SUB/1(In1)
  [EKF_lat2] -> EKF_LAT_SUB/2(In2)
  [EKF_lat1] -> EKF_LAT_SUB/3(In3)
  [EKF_lat0] -> EKF_LAT_SUB/4(In4)
  EKF_HEAD_SUB/1(EKF_HEAD) -> EKF_HEAD/1, To Workspace1/1
  [EKF_head3] -> EKF_HEAD_SUB/1(In1)
  [EKF_head2] -> EKF_HEAD_SUB/2(In2)
  [EKF_head1] -> EKF_HEAD_SUB/3(In3)
  [EKF_head0] -> EKF_HEAD_SUB/4(In4)
  EKF_LONG_SUB/1(EKF_LONG) -> [EKF_long], To Workspace29/1, EKF_LONG/1
  [EKF_long3] -> EKF_LONG_SUB/1(In1)
  [EKF_long2] -> EKF_LONG_SUB/2(In2)
  [EKF_long1] -> EKF_LONG_SUB/3(In3)
  [EKF_long0] -> EKF_LONG_SUB/4(In4)

== system GPS1_Kvaser_R2018a_v3_0719/EKF_HEAD_SUB ==
  In1 : Inport
  In2 : Inport  Port=2
  In3 : Inport  Port=3
  In4 : Inport  Port=4
  Plus8 : Sum  Inputs=++++
  EKF_HEAD : Outport
  wires:
  Plus8/1 -> EKF_HEAD/1
  In4/1 -> Plus8/4
  In2/1 -> Plus8/2
  In1/1 -> Plus8/1
  In3/1 -> Plus8/3

== system GPS1_Kvaser_R2018a_v3_0719/EKF_LAT_SUB ==
  In1 : Inport
  In2 : Inport  Port=2
  In3 : Inport  Port=3
  In4 : Inport  Port=4
  Plus7 : Sum  Inputs=++++
  EKF_LAT : Outport
  wires:
  In3/1 -> Plus7/3
  In2/1 -> Plus7/2
  Plus7/1 -> EKF_LAT/1
  In1/1 -> Plus7/1
  In4/1 -> Plus7/4

== system GPS1_Kvaser_R2018a_v3_0719/EKF_LONG_SUB ==
  In1 : Inport
  In2 : Inport  Port=2
  In3 : Inport  Port=3
  In4 : Inport  Port=4
  Plus9 : Sum  Inputs=++++
  EKF_LONG : Outport
  wires:
  In4/1 -> Plus9/4
  In3/1 -> Plus9/3
  In2/1 -> Plus9/2
  In1/1 -> Plus9/1
  Plus9/1 -> EKF_LONG/1

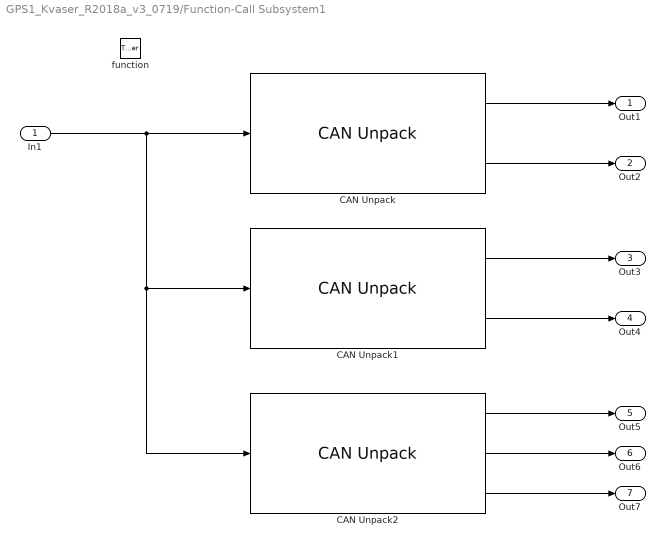
== system GPS1_Kvaser_R2018a_v3_0719/Function-Call Subsystem1 ==
  In1 : Inport
  function : TriggerPort  TriggerType=function-call  VariantControl=Variant
  CAN Unpack : canmsglib/CAN Unpack  CANdbFile=C:\Users\ZNYZY\Desktop\SYY\DBC\RAC-C1P.dbc  MsgList=(none)  MsgName=Latitude_And_Longitude  MsgIDType=Standard (11-bit identifier)  MsgIdentifier=305  MsgLength=8  SignalInfo=latitude$0$32$1$1$1$0$1.000000e-07$0$-Inf$Inf$#longitude$32$32$1$1$1$0$1.000000e-07$0$-Inf$Inf$#  IDPort=off  TimestampPort=off  ErrorPort=off  RemotePort=off  LengthPort=off  StatusPort=off  ApplyMinMax=off  NSignals=2  StartBits=str2num('[int32(0);int32(32)]')  SignalSizes=str2num('[int32(32);int32(32)]')  ByteOrders=str2num('[int32(1);int32(1)]')  DataTypes=str2num('[int32(1);int32(1)]')  MultiplexTypes=str2num('[int32(1);int32(1)]')  MultiplexValues=str2num('[double(0);double(0)]')  Factors=str2num('[double(1.000000e-07);double(1.000000e-07)]')  Offsets=str2num('[double(0);double(0)]')  Minimums=str2num('[double(-Inf);double(-Inf)]')  Maximums=str2num('[double(Inf);double(Inf)]')
      settings: SourceProductBaseCode=ME,XP,VN  DataFormat=CANdb specified signals
  CAN Unpack1 : canmsglib/CAN Unpack  CANdbFile=C:\Users\ZNYZY\Desktop\SYY\DBC\RAC-C1P.dbc  MsgList=(none)  MsgName=Position  MsgIDType=Standard (11-bit identifier)  MsgIdentifier=306  MsgLength=8  SignalInfo=altitude$0$32$1$1$1$0$1.000000e-03$0$-Inf$Inf$#heading$32$32$1$2$1$0$1.000000e-03$0$-Inf$Inf$#  IDPort=off  TimestampPort=off  ErrorPort=off  RemotePort=off  LengthPort=off  StatusPort=off  ApplyMinMax=off  NSignals=2  StartBits=str2num('[int32(0);int32(32)]')  SignalSizes=str2num('[int32(32);int32(32)]')  ByteOrders=str2num('[int32(1);int32(1)]')  DataTypes=str2num('[int32(1);int32(2)]')  MultiplexTypes=str2num('[int32(1);int32(1)]')  MultiplexValues=str2num('[double(0);double(0)]')  Factors=str2num('[double(1.000000e-03);double(1.000000e-03)]')  Offsets=str2num('[double(0);double(0)]')  Minimums=str2num('[double(-Inf);double(-Inf)]')  Maximums=str2num('[double(Inf);double(Inf)]')
      settings: SourceProductBaseCode=ME,XP,VN  DataFormat=CANdb specified signals
  CAN Unpack2 : canmsglib/CAN Unpack  CANdbFile=C:\Users\ZNYZY\Desktop\SYY\DBC\RAC-C1P.dbc  MsgList=(none)  MsgName=Vehicle_Statue  MsgIDType=Standard (11-bit identifier)  MsgIdentifier=304  MsgLength=8  SignalInfo=position_type$48$8$1$2$1$0$1$0$-Inf$Inf$#satellites$56$8$1$2$1$0$1$0$-Inf$Inf$#speed$16$32$1$1$1$0$1.000000e-02$0$-Inf$Inf$#  IDPort=off  TimestampPort=off  ErrorPort=off  RemotePort=off  LengthPort=off  StatusPort=off  ApplyMinMax=off  NSignals=3  StartBits=str2num('[int32(48);int32(56);int32(16)]')  SignalSizes=str2num('[int32(8);int32(8);int32(32)]')  ByteOrders=str2num('[int32(1);int32(1);int32(1)]')  DataTypes=str2num('[int32(2);int32(2);int32(1)]')  MultiplexTypes=str2num('[int32(1);int32(1);int32(1)]')  MultiplexValues=str2num('[double(0);double(0);double(0)]')  Factors=str2num('[double(1);double(1);double(1.000000e-02)]')  Offsets=str2num('[double(0);double(0);double(0)]')  Minimums=str2num('[double(-Inf);double(-Inf);double(-Inf)]')  Maximums=str2num('[double(Inf);double(Inf);double(Inf)]')
      settings: SourceProductBaseCode=ME,XP,VN  DataFormat=CANdb specified signals
  Out1 : Outport  VectorParamsAs1DForOutWhenUnconnected=off
  Out2 : Outport  Port=2  VectorParamsAs1DForOutWhenUnconnected=off
  Out3 : Outport  Port=3  VectorParamsAs1DForOutWhenUnconnected=off
  Out4 : Outport  Port=4  VectorParamsAs1DForOutWhenUnconnected=off
  Out5 : Outport  Port=5  VectorParamsAs1DForOutWhenUnconnected=off
  Out6 : Outport  Port=6  VectorParamsAs1DForOutWhenUnconnected=off
  Out7 : Outport  Port=7  VectorParamsAs1DForOutWhenUnconnected=off
  wires:
  CAN Unpack1/2 -> Out4/1
  CAN Unpack1/1 -> Out3/1
  CAN Unpack/2 -> Out2/1
  CAN Unpack/1 -> Out1/1
  In1/1 -> CAN Unpack/1, CAN Unpack2/1, CAN Unpack1/1
  CAN Unpack2/1 -> Out5/1
  CAN Unpack2/2 -> Out6/1
  CAN Unpack2/3 -> Out7/1

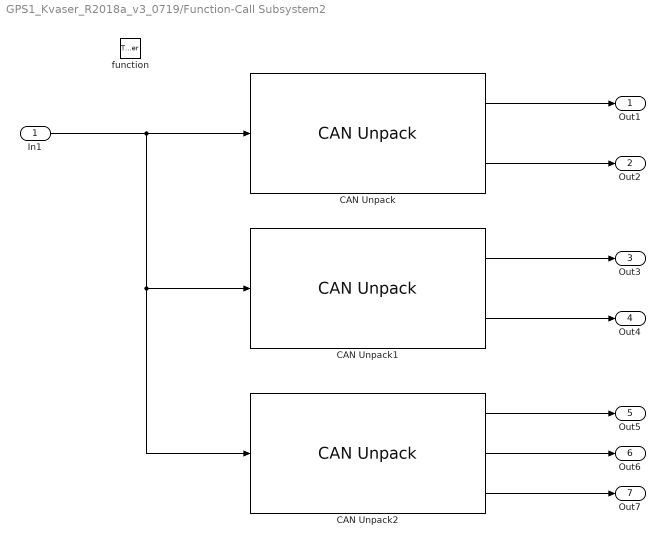
== system GPS1_Kvaser_R2018a_v3_0719/Function-Call Subsystem2 ==
  In1 : Inport
  function : TriggerPort  TriggerType=function-call  VariantControl=Variant
  CAN Unpack : canmsglib/CAN Unpack  CANdbFile=C:\Users\ZNYZY\Desktop\SYY\DBC\RAC-C1P.dbc  MsgList=(none)  MsgName=Latitude_And_Longitude  MsgIDType=Standard (11-bit identifier)  MsgIdentifier=305  MsgLength=8  SignalInfo=latitude$0$32$1$1$1$0$1.000000e-07$0$-Inf$Inf$#longitude$32$32$1$1$1$0$1.000000e-07$0$-Inf$Inf$#  IDPort=off  TimestampPort=off  ErrorPort=off  RemotePort=off  LengthPort=off  StatusPort=off  ApplyMinMax=off  NSignals=2  StartBits=str2num('[int32(0);int32(32)]')  SignalSizes=str2num('[int32(32);int32(32)]')  ByteOrders=str2num('[int32(1);int32(1)]')  DataTypes=str2num('[int32(1);int32(1)]')  MultiplexTypes=str2num('[int32(1);int32(1)]')  MultiplexValues=str2num('[double(0);double(0)]')  Factors=str2num('[double(1.000000e-07);double(1.000000e-07)]')  Offsets=str2num('[double(0);double(0)]')  Minimums=str2num('[double(-Inf);double(-Inf)]')  Maximums=str2num('[double(Inf);double(Inf)]')
      settings: SourceProductBaseCode=ME,XP,VN  DataFormat=CANdb specified signals
  CAN Unpack1 : canmsglib/CAN Unpack  CANdbFile=C:\Users\ZNYZY\Desktop\SYY\DBC\RAC-C1P.dbc  MsgList=(none)  MsgName=Position  MsgIDType=Standard (11-bit identifier)  MsgIdentifier=306  MsgLength=8  SignalInfo=altitude$0$32$1$1$1$0$1.000000e-03$0$-Inf$Inf$#heading$32$32$1$2$1$0$1.000000e-03$0$-Inf$Inf$#  IDPort=off  TimestampPort=off  ErrorPort=off  RemotePort=off  LengthPort=off  StatusPort=off  ApplyMinMax=off  NSignals=2  StartBits=str2num('[int32(0);int32(32)]')  SignalSizes=str2num('[int32(32);int32(32)]')  ByteOrders=str2num('[int32(1);int32(1)]')  DataTypes=str2num('[int32(1);int32(2)]')  MultiplexTypes=str2num('[int32(1);int32(1)]')  MultiplexValues=str2num('[double(0);double(0)]')  Factors=str2num('[double(1.000000e-03);double(1.000000e-03)]')  Offsets=str2num('[double(0);double(0)]')  Minimums=str2num('[double(-Inf);double(-Inf)]')  Maximums=str2num('[double(Inf);double(Inf)]')
      settings: SourceProductBaseCode=ME,XP,VN  DataFormat=CANdb specified signals
  CAN Unpack2 : canmsglib/CAN Unpack  CANdbFile=C:\Users\ZNYZY\Desktop\SYY\DBC\RAC-C1P.dbc  MsgList=(none)  MsgName=Vehicle_Statue  MsgIDType=Standard (11-bit identifier)  MsgIdentifier=304  MsgLength=8  SignalInfo=position_type$48$8$1$2$1$0$1$0$-Inf$Inf$#satellites$56$8$1$2$1$0$1$0$-Inf$Inf$#speed$16$32$1$1$1$0$1.000000e-02$0$-Inf$Inf$#  IDPort=off  TimestampPort=off  ErrorPort=off  RemotePort=off  LengthPort=off  StatusPort=off  ApplyMinMax=off  NSignals=3  StartBits=str2num('[int32(48);int32(56);int32(16)]')  SignalSizes=str2num('[int32(8);int32(8);int32(32)]')  ByteOrders=str2num('[int32(1);int32(1);int32(1)]')  DataTypes=str2num('[int32(2);int32(2);int32(1)]')  MultiplexTypes=str2num('[int32(1);int32(1);int32(1)]')  MultiplexValues=str2num('[double(0);double(0);double(0)]')  Factors=str2num('[double(1);double(1);double(1.000000e-02)]')  Offsets=str2num('[double(0);double(0);double(0)]')  Minimums=str2num('[double(-Inf);double(-Inf);double(-Inf)]')  Maximums=str2num('[double(Inf);double(Inf);double(Inf)]')
      settings: SourceProductBaseCode=ME,XP,VN  DataFormat=CANdb specified signals
  Out1 : Outport  VectorParamsAs1DForOutWhenUnconnected=off
  Out2 : Outport  Port=2  VectorParamsAs1DForOutWhenUnconnected=off
  Out3 : Outport  Port=3  VectorParamsAs1DForOutWhenUnconnected=off
  Out4 : Outport  Port=4  VectorParamsAs1DForOutWhenUnconnected=off
  Out5 : Outport  Port=5  VectorParamsAs1DForOutWhenUnconnected=off
  Out6 : Outport  Port=6  VectorParamsAs1DForOutWhenUnconnected=off
  Out7 : Outport  Port=7  VectorParamsAs1DForOutWhenUnconnected=off
  wires:
  CAN Unpack1/2 -> Out4/1
  CAN Unpack1/1 -> Out3/1
  CAN Unpack/2 -> Out2/1
  CAN Unpack/1 -> Out1/1
  In1/1 -> CAN Unpack/1, CAN Unpack2/1, CAN Unpack1/1
  CAN Unpack2/1 -> Out5/1
  CAN Unpack2/2 -> Out6/1
  CAN Unpack2/3 -> Out7/1

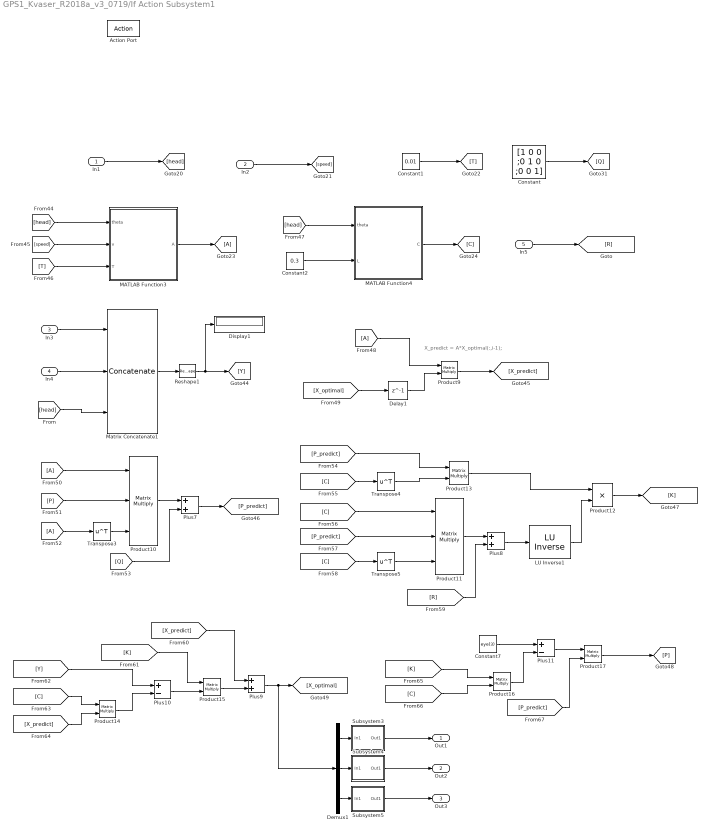
== system GPS1_Kvaser_R2018a_v3_0719/If Action Subsystem1 ==
  note: X_predict = A*X_optimal(:,i-1);
  In1 : Inport
  In2 : Inport  Port=2
  In3 : Inport  Port=3
  In4 : Inport  Port=4
  In5 : Inport  Port=5
  Action Port : ActionPort
  " LU Inverse1" : dspinverses/ LU Inverse
  Constant : Constant  Value=[1 0 0 ;0 1 0 ;0 0 1]
  Constant1 : Constant  Value=0.01
  Constant2 : Constant  Value=0.3
  Constant7 : Constant  Value=eye(3)
  Delay1 : Delay  DelayLength=1
  Demux1 : Demux  Outputs=3
  Display1 : Display
  MATLAB Function3 : MATLAB Function  TreatAsAtomicUnit=on
  MATLAB Function4 : MATLAB Function  TreatAsAtomicUnit=on
  Matrix Concatenate1 : Concatenate  NumInputs=3  Mode=Multidimensional array  ConcatenateDimension=2
  Plus10 : Sum  Inputs=+-
  Plus11 : Sum  Inputs=+-
  Plus7 : Sum
  Plus8 : Sum
  Plus9 : Sum
  Product10 : Product  Inputs=3  Multiplication=Matrix(*)
  Product11 : Product  Inputs=3  Multiplication=Matrix(*)
  Product12 : Product
  Product{9,13..17} (6 alike) : Product  Multiplication=Matrix(*)
  Reshape1 : Reshape  OutputDimensionality=Customize  OutputDimensions=[3,1]
  Subsystem3 : Subsystem
  Subsystem4 : Subsystem
  Subsystem5 : Subsystem
  Transpose3 : Math  Operator=transpose  SaturateOnIntegerOverflow=on
  Transpose4 : Math  Operator=transpose  SaturateOnIntegerOverflow=on
  Transpose5 : Math  Operator=transpose  SaturateOnIntegerOverflow=on
  Out1 : Outport
  Out2 : Outport  Port=2
  Out3 : Outport  Port=3
  wires:
  [A] -> Product10/1
  [C] -> Product11/1
  [Y] -> Plus10/1
  Plus8/1 -> " LU Inverse1"/1
  [P_predict] -> Product17/2
  [A] -> Transpose3/1
  [C] -> Product14/1
  [X_predict] -> Plus9/1
  Subsystem5/1(Out1) -> Out3/1
  [C] -> Product16/2
  Subsystem3/1(Out1) -> Out1/1
  Reshape1/1 -> [Y], Display1/1
  Product16/1 -> Plus11/2
  [P] -> Product10/2
  [C] -> Transpose4/1
  Demux1/3 -> Subsystem5/1(In1)
  Product11/1 -> Plus8/1
  [P_predict] -> Product11/2
  [T] -> MATLAB Function3/3(T)
  Demux1/2 -> Subsystem4/1(In1)
  Plus9/1 -> Demux1/1, [X_optimal]
  Product14/1 -> Plus10/2
  Product17/1 -> [P]
  [C] -> Transpose5/1
  [head] -> MATLAB Function3/1(theta)
  In4/1 -> Matrix Concatenate1/2
  [head] -> Matrix Concatenate1/3
  Product13/1 -> Product12/1
  In5/1 -> [R]
  [K] -> Product15/1
  [Q] -> Plus7/2
  Transpose4/1 -> Product13/2
  Transpose5/1 -> Product11/3
  Plus7/1 -> [P_predict]
  Matrix Concatenate1/1 -> Reshape1/1
  [A] -> Product9/1
  Constant7/1 -> Plus11/1
  Product9/1 -> [X_predict]
  MATLAB Function4/1(C) -> [C]
  Product12/1 -> [K]
  [head] -> MATLAB Function4/1(theta)
  [R] -> Plus8/2
  Subsystem4/1(Out1) -> Out2/1
  Constant1/1 -> [T]
  Product15/1 -> Plus9/2
  Constant/1 -> [Q]
  Plus10/1 -> Product15/2
  [X_predict] -> Product14/2
  In2/1 -> [speed]
  In1/1 -> [head]
  Transpose3/1 -> Product10/3
  [K] -> Product16/1
  Demux1/1 -> Subsystem3/1(In1)
  " LU Inverse1"/1 -> Product12/2
  In3/1 -> Matrix Concatenate1/1
  Plus11/1 -> Product17/1
  Constant2/1 -> MATLAB Function4/2(L)
  [P_predict] -> Product13/1
  Product10/1 -> Plus7/1
  MATLAB Function3/1(A) -> [A]
  [speed] -> MATLAB Function3/2(v)
  Delay1/1 -> Product9/2
  [X_optimal] -> Delay1/1

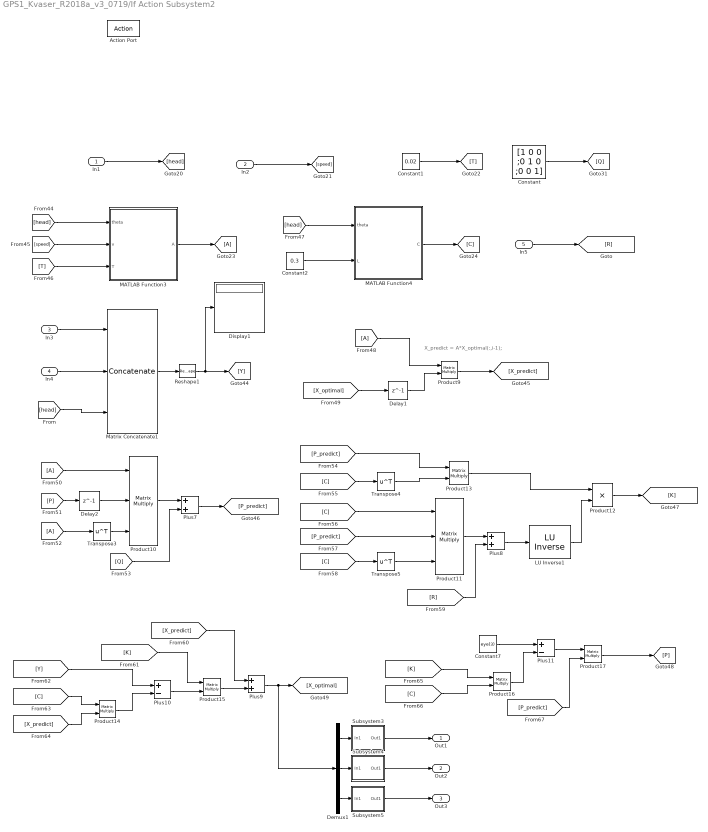
== system GPS1_Kvaser_R2018a_v3_0719/If Action Subsystem2 ==
  note: X_predict = A*X_optimal(:,i-1);
  In1 : Inport
  In2 : Inport  Port=2
  In3 : Inport  Port=3
  In4 : Inport  Port=4
  In5 : Inport  Port=5
  Action Port : ActionPort
  " LU Inverse1" : dspinverses/ LU Inverse
  Constant : Constant  Value=[1 0 0 ;0 1 0 ;0 0 1]
  Constant1 : Constant  Value=0.02
  Constant2 : Constant  Value=0.3
  Constant7 : Constant  Value=eye(3)
  Delay1 : Delay  DelayLength=1
  Delay2 : Delay  DelayLength=1
  Demux1 : Demux  Outputs=3
  Display1 : Display
  MATLAB Function3 : MATLAB Function  TreatAsAtomicUnit=on
  MATLAB Function4 : MATLAB Function  TreatAsAtomicUnit=on
  Matrix Concatenate1 : Concatenate  NumInputs=3  Mode=Multidimensional array  ConcatenateDimension=2
  Plus10 : Sum  Inputs=+-
  Plus11 : Sum  Inputs=+-
  Plus7 : Sum
  Plus8 : Sum
  Plus9 : Sum
  Product10 : Product  Inputs=3  Multiplication=Matrix(*)
  Product11 : Product  Inputs=3  Multiplication=Matrix(*)
  Product12 : Product
  Product{9,13..17} (6 alike) : Product  Multiplication=Matrix(*)
  Reshape1 : Reshape  OutputDimensionality=Customize  OutputDimensions=[3,1]
  Subsystem3 : Subsystem
  Subsystem4 : Subsystem
  Subsystem5 : Subsystem
  Transpose3 : Math  Operator=transpose  SaturateOnIntegerOverflow=on
  Transpose4 : Math  Operator=transpose  SaturateOnIntegerOverflow=on
  Transpose5 : Math  Operator=transpose  SaturateOnIntegerOverflow=on
  Out1 : Outport
  Out2 : Outport  Port=2
  Out3 : Outport  Port=3
  wires:
  [A] -> Product10/1
  [C] -> Product11/1
  [Y] -> Plus10/1
  Plus8/1 -> " LU Inverse1"/1
  [P_predict] -> Product17/2
  [A] -> Transpose3/1
  [C] -> Product14/1
  [X_predict] -> Plus9/1
  Subsystem5/1(Out1) -> Out3/1
  [C] -> Product16/2
  Subsystem3/1(Out1) -> Out1/1
  Reshape1/1 -> [Y], Display1/1
  Product16/1 -> Plus11/2
  [P] -> Delay2/1
  [C] -> Transpose4/1
  Demux1/3 -> Subsystem5/1(In1)
  Product11/1 -> Plus8/1
  [P_predict] -> Product11/2
  [T] -> MATLAB Function3/3(T)
  Demux1/2 -> Subsystem4/1(In1)
  Plus9/1 -> Demux1/1, [X_optimal]
  Product14/1 -> Plus10/2
  Product17/1 -> [P]
  [C] -> Transpose5/1
  [head] -> MATLAB Function3/1(theta)
  In4/1 -> Matrix Concatenate1/2
  [head] -> Matrix Concatenate1/3
  Product13/1 -> Product12/1
  In5/1 -> [R]
  [K] -> Product15/1
  [Q] -> Plus7/2
  Transpose4/1 -> Product13/2
  Transpose5/1 -> Product11/3
  Plus7/1 -> [P_predict]
  Matrix Concatenate1/1 -> Reshape1/1
  [A] -> Product9/1
  Constant7/1 -> Plus11/1
  Product9/1 -> [X_predict]
  MATLAB Function4/1(C) -> [C]
  Product12/1 -> [K]
  [head] -> MATLAB Function4/1(theta)
  [R] -> Plus8/2
  Subsystem4/1(Out1) -> Out2/1
  Constant1/1 -> [T]
  Product15/1 -> Plus9/2
  Constant/1 -> [Q]
  Plus10/1 -> Product15/2
  [X_predict] -> Product14/2
  In2/1 -> [speed]
  In1/1 -> [head]
  Transpose3/1 -> Product10/3
  [K] -> Product16/1
  Demux1/1 -> Subsystem3/1(In1)
  " LU Inverse1"/1 -> Product12/2
  In3/1 -> Matrix Concatenate1/1
  Plus11/1 -> Product17/1
  Constant2/1 -> MATLAB Function4/2(L)
  [P_predict] -> Product13/1
  Product10/1 -> Plus7/1
  MATLAB Function3/1(A) -> [A]
  [speed] -> MATLAB Function3/2(v)
  Delay1/1 -> Product9/2
  [X_optimal] -> Delay1/1
  Delay2/1 -> Product10/2

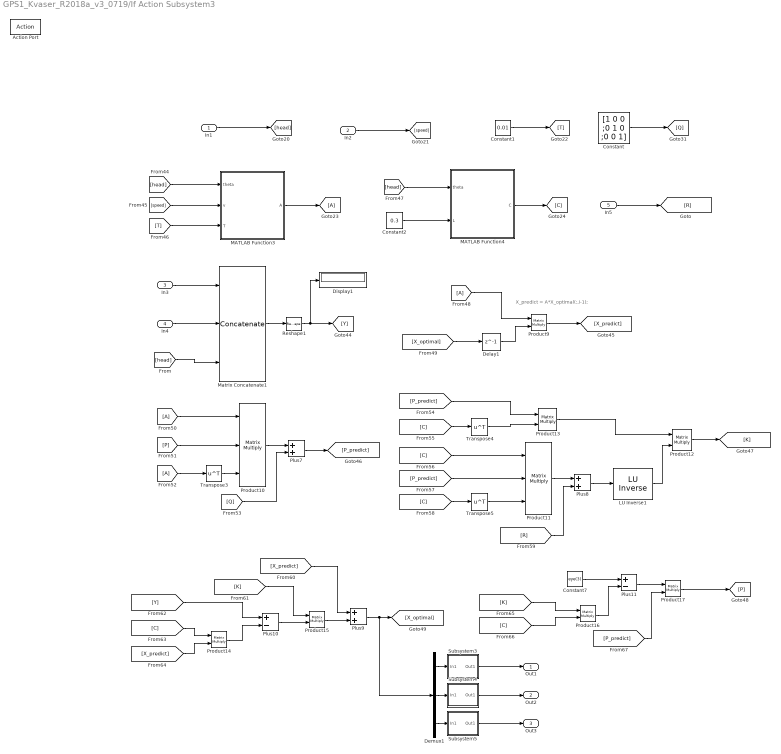
== system GPS1_Kvaser_R2018a_v3_0719/If Action Subsystem3 ==
  note: X_predict = A*X_optimal(:,i-1);
  In1 : Inport
  In2 : Inport  Port=2
  In3 : Inport  Port=3
  In4 : Inport  Port=4
  In5 : Inport  Port=5
  Action Port : ActionPort
  " LU Inverse1" : dspinverses/ LU Inverse
  Constant : Constant  Value=[1 0 0 ;0 1 0 ;0 0 1]
  Constant1 : Constant  Value=0.01
  Constant2 : Constant  Value=0.3
  Constant7 : Constant  Value=eye(3)
  Delay1 : Delay  DelayLength=1
  Demux1 : Demux  Outputs=3
  Display1 : Display
  MATLAB Function3 : MATLAB Function  TreatAsAtomicUnit=on
  MATLAB Function4 : MATLAB Function  TreatAsAtomicUnit=on
  Matrix Concatenate1 : Concatenate  NumInputs=3  Mode=Multidimensional array  ConcatenateDimension=2
  Plus10 : Sum  Inputs=+-
  Plus11 : Sum  Inputs=+-
  Plus7 : Sum
  Plus8 : Sum
  Plus9 : Sum
  Product10 : Product  Inputs=3  Multiplication=Matrix(*)
  Product11 : Product  Inputs=3  Multiplication=Matrix(*)
  Product{9,12..17} (7 alike) : Product  Multiplication=Matrix(*)
  Reshape1 : Reshape  OutputDimensionality=Customize  OutputDimensions=[3,1]
  Subsystem3 : Subsystem
  Subsystem4 : Subsystem
  Subsystem5 : Subsystem
  Transpose3 : Math  Operator=transpose  SaturateOnIntegerOverflow=on
  Transpose4 : Math  Operator=transpose  SaturateOnIntegerOverflow=on
  Transpose5 : Math  Operator=transpose  SaturateOnIntegerOverflow=on
  Out1 : Outport
  Out2 : Outport  Port=2
  Out3 : Outport  Port=3
  wires:
  [head] -> MATLAB Function4/1(theta)
  Constant1/1 -> [T]
  [speed] -> MATLAB Function3/2(v)
  Subsystem5/1(Out1) -> Out3/1
  [head] -> MATLAB Function3/1(theta)
  Subsystem4/1(Out1) -> Out2/1
  [head] -> Matrix Concatenate1/3
  MATLAB Function3/1(A) -> [A]
  Subsystem3/1(Out1) -> Out1/1
  In4/1 -> Matrix Concatenate1/2
  Product9/1 -> [X_predict]
  [P_predict] -> Product11/2
  [K] -> Product15/1
  Product15/1 -> Plus9/2
  [X_optimal] -> Delay1/1
  [C] -> Product16/2
  Product13/1 -> Product12/1
  Demux1/3 -> Subsystem5/1(In1)
  [C] -> Transpose4/1
  Product12/1 -> [K]
  Transpose3/1 -> Product10/3
  [C] -> Transpose5/1
  [Y] -> Plus10/1
  Product17/1 -> [P]
  Matrix Concatenate1/1 -> Reshape1/1
  [A] -> Transpose3/1
  Transpose4/1 -> Product13/2
  In1/1 -> [head]
  Plus7/1 -> [P_predict]
  [A] -> Product9/1
  In5/1 -> [R]
  [C] -> Product11/1
  Constant2/1 -> MATLAB Function4/2(L)
  MATLAB Function4/1(C) -> [C]
  " LU Inverse1"/1 -> Product12/2
  Transpose5/1 -> Product11/3
  [X_predict] -> Product14/2
  Delay1/1 -> Product9/2
  Plus8/1 -> " LU Inverse1"/1
  [A] -> Product10/1
  Plus10/1 -> Product15/2
  Product11/1 -> Plus8/1
  [K] -> Product16/1
  [R] -> Plus8/2
  [P_predict] -> Product17/2
  [Q] -> Plus7/2
  [P_predict] -> Product13/1
  [C] -> Product14/1
  In2/1 -> [speed]
  Demux1/1 -> Subsystem3/1(In1)
  Reshape1/1 -> [Y], Display1/1
  [X_predict] -> Plus9/1
  Plus9/1 -> Demux1/1, [X_optimal]
  In3/1 -> Matrix Concatenate1/1
  Product14/1 -> Plus10/2
  Constant7/1 -> Plus11/1
  [T] -> MATLAB Function3/3(T)
  Product16/1 -> Plus11/2
  Plus11/1 -> Product17/1
  [P] -> Product10/2
  Demux1/2 -> Subsystem4/1(In1)
  Constant/1 -> [Q]
  Product10/1 -> Plus7/1
